simulink model "hdv_hydroelectropowertrain_model"  (R2026a)
settings: Solver=ode1be  StopTime=simulation_length  FixedStep=tsample  MaxStep=tsample
undefined symbols (not defined in the file): alpha, Apump, available_torque, Bpump, btheta_shaft, C1, consumption, Cpump, dp_lim, E0, E1, E2, E3, E_1, Elog, eta_v_m, eta_v_p, ki_dp_comp, ki_te_comp, kp_ctrl_m, kp_dp_comp, kp_te_comp, Kpump, load_blade_enable, Lpump, M, magnitude, Ncell, Npump, omega_e_rpm_ref, omega_l_max_rpm, q1Kalman, q2Kalman, q3Kalman, Qhr, R0, R1, R_tg, rKalman, rpm_base, rpm_consumption, simulation_length, tau_load, tau_load_max, Tc, torque_base, torque_consumption, torque_friction_base, tsample, v_track1_ref, v_track2_ref, valve_mmorifice_max, xv_m_max
libraries: fl_lib x383, nesl_utility x162, linear_swashplate_ctrl_lib x8, flexshaft_lib x5, bichamber_piston_lib x5, variable_displacement_motor_lib x4, variable_displacement_pump_lib x4, fixed_displacement_pump_lib x4, relief_valve_lib x4, inverse_shuttle_valve_lib x4, hydrostatic_threeway_valve_bichamber_piston_lib x4, hydrostatic_fourway_valve_bichamber_piston_lib x4
(part 7 of 8)

== system hdv_hydroelectropowertrain_model/PR776_powertrain/Hydrostatic_powertrain/driveine_RD1/vd_ctrl_pump_RD/hose3 ==
  Constant Area Hydraulic Orifice : fl_lib/Hydraulic/Hydraulic Elements/Constant Area Hydraulic Orifice  area=1e-8 m^2  C_d=0.7  lam_spec=1  B_lam=0.999  Re_cr=12  q_specify=off  q_priority=None  q=0.001 m^3/s  q_nominal_specify=off  q_nominal_value=1  q_nominal_unit=m^3/s  p_specify=off  p_priority=None  p=0 Pa  p_nominal_specify=off  p_nominal_value=1  p_nominal_unit=Pa
  Constant Area Hydraulic Orifice1 : fl_lib/Hydraulic/Hydraulic Elements/Constant Area Hydraulic Orifice  area=1e-8 m^2  C_d=0.7  lam_spec=1  B_lam=0.999  Re_cr=12  q_specify=off  q_priority=None  q=0.001 m^3/s  q_nominal_specify=off  q_nominal_value=1  q_nominal_unit=m^3/s  p_specify=off  p_priority=None  p=0 Pa  p_nominal_specify=off  p_nominal_value=1  p_nominal_unit=Pa
  Hydraulic Flow Rate Sensor3 : fl_lib/Hydraulic/Hydraulic Sensors/Hydraulic Flow Rate Sensor
  Hydraulic Flow Rate Source : fl_lib/Hydraulic/Hydraulic Sources/Hydraulic Flow Rate Source
  Hydraulic Pressure Sensor2 : fl_lib/Hydraulic/Hydraulic Sensors/Hydraulic Pressure Sensor
  Hydraulic Pressure Source : fl_lib/Hydraulic/Hydraulic Sources/Hydraulic Pressure Source
  Hydraulic Reference : fl_lib/Hydraulic/Hydraulic Elements/Hydraulic Reference
  PS Gain : fl_lib/Physical Signals/Functions/PS Gain  gain=1 Pa
  PS Gain1 : fl_lib/Physical Signals/Functions/PS Gain  gain=1 Pa^-1
  PS Gain2 : fl_lib/Physical Signals/Functions/PS Gain  gain=1 m^3/s
  PS Gain3 : fl_lib/Physical Signals/Functions/PS Gain  gain=1 m^-3*s
  PS Transfer Function : fl_lib/Physical Signals/Linear Operators/PS Transfer Function  transfer_function_type=foundation.enum.transfer_function_type.lag  T=0.01 s  T1=2 s  T2=1 s  reset_method=foundation.enum.IntegratorResetSpec.None  initial_condition_spec=foundation.enum.IntegratorICSpec.Internal  y0=0
  PS Transfer Function1 : fl_lib/Physical Signals/Linear Operators/PS Transfer Function  transfer_function_type=foundation.enum.transfer_function_type.lag  T=0.01 s  T1=2 s  T2=1 s  reset_method=foundation.enum.IntegratorResetSpec.None  initial_condition_spec=foundation.enum.IntegratorICSpec.Internal  y0=0
  A : PMIOPort  Side=Left
  AA : PMIOPort  Port=2  Side=Right
  B : PMIOPort  Port=3  Side=Left
  BB : PMIOPort  Port=4  Side=Right
  connections:
  AA/RConn1 -- Constant Area Hydraulic Orifice1/LConn1 -- Hydraulic Flow Rate Sensor3/RConn2
  PS Gain2/RConn1 -- Hydraulic Flow Rate Source/RConn1
  Hydraulic Flow Rate Sensor3/RConn1 -- PS Gain3/LConn1
  Hydraulic Flow Rate Sensor3/LConn1 -- Hydraulic Pressure Source/LConn1
  Hydraulic Pressure Source/RConn1 -- PS Gain/RConn1
  PS Gain1/LConn1 -- Hydraulic Pressure Sensor2/RConn2
  Hydraulic Pressure Source/RConn2 -- Hydraulic Pressure Sensor2/RConn1 -- Constant Area Hydraulic Orifice/RConn1 -- B/RConn1 -- Hydraulic Flow Rate Source/LConn1 -- Constant Area Hydraulic Orifice1/RConn1 -- Hydraulic Reference/LConn1 -- BB/RConn1
  PS Transfer Function1/RConn1 -- PS Gain2/LConn1
  PS Transfer Function/RConn1 -- PS Gain/LConn1
  A/RConn1 -- Constant Area Hydraulic Orifice/LConn1 -- Hydraulic Pressure Sensor2/LConn1 -- Hydraulic Flow Rate Source/RConn2
  PS Gain3/RConn1 -- PS Transfer Function1/LConn1
  PS Gain1/RConn1 -- PS Transfer Function/LConn1

== system hdv_hydroelectropowertrain_model/PR776_powertrain/Hydrostatic_powertrain/driveine_RD1/vd_ctrl_pump_RD/servo pump RD ==
  displacement reference pu : Inport
  Gain : Gain  Gain=0.03647/2
  PS Gain : fl_lib/Physical Signals/Functions/PS Gain  gain=1/(0.03647/2) m^-1
  PS-Simulink Converter7 : nesl_utility/PS-Simulink Converter  PhysicalDomain=network_engine_domain  SubClassName=ps_output  LeftPortType=input  RightPortType=output  PseudoPeriodic=off  Frequencies=[]  VectorFormat=1-D array  Unit=1  AffineConversion=off
  hydrostatic_fourway_valve_bichamber : hydrostatic_fourway_valve_bichamber_piston_lib/hydrostatic_fourway_valve_bichamber  D1=D1 m  D2=D2 m  Lp=Lp m  xv_max=xv_max mm  mp=mp kg  kp=kp N/m  bp=bp N/(m/s)  q1_specify=off  q1_priority=None  q1=0 m^3/s  q1_nominal_specify=off  q1_nominal_unit=m^3/s  q1_nominal_value=1  q2_specify=off  q2_priority=None  q2=0 m^3/s  q2_nominal_specify=off  q2_nominal_unit=m^3/s  q2_nominal_value=1  qin_specify=off  qin_priority=None  qin=0 m^3/s  qin_nominal_specify=off  qin_nominal_unit=m^3/s  qin_nominal_value=1  qout_specify=off  qout_priority=None  qout=0 m^3/s  qout_nominal_specify=off  qout_nominal_unit=m^3/s  qout_nominal_value=1  p1_specify=off  p1_priority=High  p1=125 bar  p1_nominal_specify=off  p1_nominal_unit=bar  p1_nominal_value=1  p2_specify=off  p2_priority=High  p2=125 bar  p2_nominal_specify=off  p2_nominal_unit=bar  p2_nominal_value=1  fp_specify=off  fp_priority=None  fp=0 N  fp_nominal_specify=off  fp_nominal_unit=N  fp_nominal_value=1  vp_specify=off  vp_priority=None  vp=0 m/s  vp_nominal_specify=off  vp_nominal_unit=m/s  vp_nominal_value=1  xp_specify=off  xp_priority=High  xp=500 mm  xp_nominal_specify=off  xp_nominal_unit=mm  xp_nominal_value=1
  pmlinear_actuator : pm_linear_actuator_lib/pmlinear_actuator  Bm=1 s*V/m^2  mv=mv kg  Lc=Lc H  Rc=Rc Ohm  bv=bv N/(m/s)  h=h m  xv_max=xv_max mm  n=n  ic_specify=off  ic_priority=High  ic=0 A  ic_nominal_specify=off  ic_nominal_unit=A  ic_nominal_value=1  vv_specify=off  vv_priority=None  vv=0 m/s  vv_nominal_specify=off  vv_nominal_unit=m/s  vv_nominal_value=1  xv_specify=off  xv_priority=None  xv=0 m  xv_nominal_specify=off  xv_nominal_unit=m  xv_nominal_value=1
  servo_ctrl : Subsystem
  pS : PMIOPort  Side=Left
  pT : PMIOPort  Port=2  Side=Left
  vd pu : PMIOPort  Port=3  Side=Right
  wires:
  Gain/1 -> servo_ctrl/1(ref)
  PS-Simulink Converter7/1 -> servo_ctrl/2(xp)  "xp"
  displacement reference pu/1 -> Gain/1
  connections:
  hydrostatic_fourway_valve_bichamber/LConn3 -- pT/RConn1
  hydrostatic_fourway_valve_bichamber/LConn2 -- pS/RConn1
  hydrostatic_fourway_valve_bichamber/RConn2 -- PS Gain/LConn1 -- PS-Simulink Converter7/LConn1
  servo_ctrl/RConn1 -- pmlinear_actuator/LConn1
  pmlinear_actuator/RConn1 -- hydrostatic_fourway_valve_bichamber/LConn1
  PS Gain/RConn1 -- vd pu/RConn1

== system hdv_hydroelectropowertrain_model/PR776_powertrain/Hydrostatic_powertrain/driveline_RD2/pressure_charge_system_RD/Subsystem ==
  Fixed displacement pump : fixed_displacement_pump_lib/Fixed displacement pump  max_Dv=27 cm^3/rev  inertia_pump=0.05 kg*m^2  oil_vol=2.0 l  bp=0.0025 N*m/(rad/s)  lk=1e-6 m  t_specify=off  t_priority=None  t=0 N*m  t_nominal_specify=off  t_nominal_unit=N*m  t_nominal_value=1  q_specify=off  q_priority=None  q=0 m^3/s  q_nominal_specify=off  q_nominal_unit=m^3/s  q_nominal_value=1  qt_specify=off  qt_priority=None  qt=0 m^3/s  qt_nominal_specify=off  qt_nominal_unit=m^3/s  qt_nominal_value=1  qleak_specify=off  qleak_priority=None  qleak=0 m^3/s  qleak_nominal_specify=off  qleak_nominal_unit=m^3/s  qleak_nominal_value=1  Dv_specify=off  Dv_priority=None  Dv=0 cm^3  Dv_nominal_specify=off  Dv_nominal_unit=cm^3  Dv_nominal_value=1  dp_specify=off  dp_priority=None  dp=0 Pa  dp_nominal_specify=off  dp_nominal_unit=Pa  dp_nominal_value=1  we_specify=off  we_priority=None  we=0 rad/s  we_nominal_specify=off  we_nominal_unit=rad/s  we_nominal_value=1
  Hydraulic Reference3 : fl_lib/Hydraulic/Hydraulic Elements/Hydraulic Reference
  Hydraulic Reference4 : fl_lib/Hydraulic/Hydraulic Elements/Hydraulic Reference
  relief valve : relief_valve_lib/relief valve  dp_ref=32 bar  pnom=32 bar  p_set=32 bar  p_reg=12 bar  x_rv_max=12.0 mm  qA_specify=off  qA_priority=None  qA=0 m^3/s  qA_nominal_specify=off  qA_nominal_value=1  qA_nominal_unit=m^3/s  qB_specify=off  qB_priority=None  qB=0 m^3/s  qB_nominal_specify=off  qB_nominal_value=1  qB_nominal_unit=m^3/s  dp_specify=off  dp_priority=None  dp=0 Pa  dp_nominal_specify=off  dp_nominal_value=1  dp_nominal_unit=Pa  x_rv_specify=off  x_rv_priority=None  x_rv=0 m  x_rv_nominal_specify=off  x_rv_nominal_value=1  x_rv_nominal_unit=m  x_rv_flt_specify=off  x_rv_flt_priority=None  x_rv_flt=0 m  x_rv_flt_nominal_specify=off  x_rv_flt_nominal_value=1  x_rv_flt_nominal_unit=m
      settings: LogSimulationData=on
  ps : PMIOPort  Side=Right
  D : PMIOPort  Port=2  Side=Left
  connections:
  Fixed displacement pump/LConn1 -- D/RConn1
  Fixed displacement pump/RConn2 -- Hydraulic Reference3/LConn1
  Hydraulic Reference4/LConn1 -- relief valve/RConn1
  relief valve/LConn1 -- ps/RConn1 -- Fixed displacement pump/RConn1

== system hdv_hydroelectropowertrain_model/PR776_powertrain/Hydrostatic_powertrain/driveline_RD2/pressure_charge_system_RD/hydro_check_valve1 ==
  Constant Area Hydraulic Orifice5 : fl_lib/Hydraulic/Hydraulic Elements/Constant Area Hydraulic Orifice  area=1e-4 mm^2  C_d=1  lam_spec=1  B_lam=0.999  Re_cr=12  q_specify=off  q_priority=None  q=0.001 m^3/s  q_nominal_specify=off  q_nominal_value=1  q_nominal_unit=m^3/s  p_specify=off  p_priority=None  p=0 Pa  p_nominal_specify=off  p_nominal_value=1  p_nominal_unit=Pa
  Constant Area Hydraulic Orifice6 : fl_lib/Hydraulic/Hydraulic Elements/Constant Area Hydraulic Orifice  area=4 mm^2  C_d=1  lam_spec=1  B_lam=0.999  Re_cr=12  q_specify=off  q_priority=None  q=0.001 m^3/s  q_nominal_specify=off  q_nominal_value=1  q_nominal_unit=m^3/s  p_specify=off  p_priority=None  p=0 Pa  p_nominal_specify=off  p_nominal_value=1  p_nominal_unit=Pa
  Hydraulic Flow Rate Sensor : fl_lib/Hydraulic/Hydraulic Sensors/Hydraulic Flow Rate Sensor
  Hydraulic Flow Rate Source : fl_lib/Hydraulic/Hydraulic Sources/Hydraulic Flow Rate Source
  Hydraulic Pressure Sensor : fl_lib/Hydraulic/Hydraulic Sensors/Hydraulic Pressure Sensor
  Hydraulic Pressure Source2 : fl_lib/Hydraulic/Hydraulic Sources/Hydraulic Pressure Source
  Hydraulic Reference : fl_lib/Hydraulic/Hydraulic Elements/Hydraulic Reference
  PS Saturation : fl_lib/Physical Signals/Nonlinear Operators/PS Saturation  upper_limit=inf m^3/s  lower_limit=0 m^3/s  ZeroCross=true
  PS Saturation1 : fl_lib/Physical Signals/Nonlinear Operators/PS Saturation  upper_limit=inf Pa  lower_limit=0 Pa  ZeroCross=true
  PS Transfer Function : fl_lib/Physical Signals/Linear Operators/PS Transfer Function  transfer_function_type=foundation.enum.transfer_function_type.lag  T=tsample s  T1=2 s  T2=1 s  reset_method=foundation.enum.IntegratorResetSpec.None  initial_condition_spec=foundation.enum.IntegratorICSpec.Internal  y0=0 m^3/s
  PS Transfer Function1 : fl_lib/Physical Signals/Linear Operators/PS Transfer Function  transfer_function_type=foundation.enum.transfer_function_type.lag  T=tsample s  T1=2 s  T2=1 s  reset_method=foundation.enum.IntegratorResetSpec.None  initial_condition_spec=foundation.enum.IntegratorICSpec.Internal  y0=0 Pa
  A : PMIOPort  Side=Left
  B : PMIOPort  Port=2  Side=Right
  connections:
  PS Transfer Function/LConn1 -- PS Saturation/RConn1
  PS Saturation1/RConn1 -- PS Transfer Function1/LConn1
  PS Transfer Function/RConn1 -- Hydraulic Flow Rate Source/RConn1
  Constant Area Hydraulic Orifice5/LConn1 -- A/RConn1 -- Hydraulic Pressure Sensor/LConn1 -- Hydraulic Flow Rate Source/RConn2
  Hydraulic Pressure Sensor/RConn2 -- PS Saturation1/LConn1
  PS Transfer Function1/RConn1 -- Hydraulic Pressure Source2/RConn1
  PS Saturation/LConn1 -- Hydraulic Flow Rate Sensor/RConn1
  B/RConn1 -- Constant Area Hydraulic Orifice5/RConn1 -- Hydraulic Pressure Sensor/RConn1 -- Hydraulic Flow Rate Source/LConn1
  Hydraulic Pressure Source2/LConn1 -- Hydraulic Flow Rate Sensor/LConn1
  Hydraulic Pressure Source2/RConn2 -- Hydraulic Reference/LConn1 -- Constant Area Hydraulic Orifice6/RConn1
  Hydraulic Flow Rate Sensor/RConn2 -- Constant Area Hydraulic Orifice6/LConn1

== system hdv_hydroelectropowertrain_model/PR776_powertrain/Hydrostatic_powertrain/driveline_RD2/pressure_charge_system_RD/hydro_check_valve2 ==
  Constant Area Hydraulic Orifice5 : fl_lib/Hydraulic/Hydraulic Elements/Constant Area Hydraulic Orifice  area=1e-4 mm^2  C_d=1  lam_spec=1  B_lam=0.999  Re_cr=12  q_specify=off  q_priority=None  q=0.001 m^3/s  q_nominal_specify=off  q_nominal_value=1  q_nominal_unit=m^3/s  p_specify=off  p_priority=None  p=0 Pa  p_nominal_specify=off  p_nominal_value=1  p_nominal_unit=Pa
  Constant Area Hydraulic Orifice6 : fl_lib/Hydraulic/Hydraulic Elements/Constant Area Hydraulic Orifice  area=4 mm^2  C_d=1  lam_spec=1  B_lam=0.999  Re_cr=12  q_specify=off  q_priority=None  q=0.001 m^3/s  q_nominal_specify=off  q_nominal_value=1  q_nominal_unit=m^3/s  p_specify=off  p_priority=None  p=0 Pa  p_nominal_specify=off  p_nominal_value=1  p_nominal_unit=Pa
  Hydraulic Flow Rate Sensor : fl_lib/Hydraulic/Hydraulic Sensors/Hydraulic Flow Rate Sensor
  Hydraulic Flow Rate Source : fl_lib/Hydraulic/Hydraulic Sources/Hydraulic Flow Rate Source
  Hydraulic Pressure Sensor : fl_lib/Hydraulic/Hydraulic Sensors/Hydraulic Pressure Sensor
  Hydraulic Pressure Source2 : fl_lib/Hydraulic/Hydraulic Sources/Hydraulic Pressure Source
  Hydraulic Reference : fl_lib/Hydraulic/Hydraulic Elements/Hydraulic Reference
  PS Saturation : fl_lib/Physical Signals/Nonlinear Operators/PS Saturation  upper_limit=inf m^3/s  lower_limit=0 m^3/s  ZeroCross=true
  PS Saturation1 : fl_lib/Physical Signals/Nonlinear Operators/PS Saturation  upper_limit=inf Pa  lower_limit=0 Pa  ZeroCross=true
  PS Transfer Function : fl_lib/Physical Signals/Linear Operators/PS Transfer Function  transfer_function_type=foundation.enum.transfer_function_type.lag  T=tsample s  T1=2 s  T2=1 s  reset_method=foundation.enum.IntegratorResetSpec.None  initial_condition_spec=foundation.enum.IntegratorICSpec.Internal  y0=0 m^3/s
  PS Transfer Function1 : fl_lib/Physical Signals/Linear Operators/PS Transfer Function  transfer_function_type=foundation.enum.transfer_function_type.lag  T=tsample s  T1=2 s  T2=1 s  reset_method=foundation.enum.IntegratorResetSpec.None  initial_condition_spec=foundation.enum.IntegratorICSpec.Internal  y0=0 Pa
  A : PMIOPort  Side=Left
  B : PMIOPort  Port=2  Side=Right
  connections:
  Hydraulic Flow Rate Sensor/RConn2 -- Constant Area Hydraulic Orifice6/LConn1
  Constant Area Hydraulic Orifice6/RConn1 -- Hydraulic Reference/LConn1 -- Hydraulic Pressure Source2/RConn2
  Hydraulic Pressure Source2/LConn1 -- Hydraulic Flow Rate Sensor/LConn1
  Hydraulic Flow Rate Source/LConn1 -- Hydraulic Pressure Sensor/RConn1 -- Constant Area Hydraulic Orifice5/RConn1 -- B/RConn1
  PS Saturation/LConn1 -- Hydraulic Flow Rate Sensor/RConn1
  PS Transfer Function1/RConn1 -- Hydraulic Pressure Source2/RConn1
  Hydraulic Pressure Sensor/RConn2 -- PS Saturation1/LConn1
  Hydraulic Flow Rate Source/RConn2 -- Hydraulic Pressure Sensor/LConn1 -- A/RConn1 -- Constant Area Hydraulic Orifice5/LConn1
  PS Transfer Function/RConn1 -- Hydraulic Flow Rate Source/RConn1
  PS Saturation1/RConn1 -- PS Transfer Function1/LConn1
  PS Transfer Function/LConn1 -- PS Saturation/RConn1

== system hdv_hydroelectropowertrain_model/PR776_powertrain/Hydrostatic_powertrain/driveline_RD2/vd_ctrl_motor_RD/hose3 ==
  Constant Area Hydraulic Orifice : fl_lib/Hydraulic/Hydraulic Elements/Constant Area Hydraulic Orifice  area=1e-8 m^2  C_d=0.7  lam_spec=1  B_lam=0.999  Re_cr=12  q_specify=off  q_priority=None  q=0.001 m^3/s  q_nominal_specify=off  q_nominal_value=1  q_nominal_unit=m^3/s  p_specify=off  p_priority=None  p=0 Pa  p_nominal_specify=off  p_nominal_value=1  p_nominal_unit=Pa
  Constant Area Hydraulic Orifice1 : fl_lib/Hydraulic/Hydraulic Elements/Constant Area Hydraulic Orifice  area=1e-8 m^2  C_d=0.7  lam_spec=1  B_lam=0.999  Re_cr=12  q_specify=off  q_priority=None  q=0.001 m^3/s  q_nominal_specify=off  q_nominal_value=1  q_nominal_unit=m^3/s  p_specify=off  p_priority=None  p=0 Pa  p_nominal_specify=off  p_nominal_value=1  p_nominal_unit=Pa
  Hydraulic Flow Rate Sensor3 : fl_lib/Hydraulic/Hydraulic Sensors/Hydraulic Flow Rate Sensor
  Hydraulic Flow Rate Source : fl_lib/Hydraulic/Hydraulic Sources/Hydraulic Flow Rate Source
  Hydraulic Pressure Sensor2 : fl_lib/Hydraulic/Hydraulic Sensors/Hydraulic Pressure Sensor
  Hydraulic Pressure Source : fl_lib/Hydraulic/Hydraulic Sources/Hydraulic Pressure Source
  Hydraulic Reference : fl_lib/Hydraulic/Hydraulic Elements/Hydraulic Reference
  PS Gain : fl_lib/Physical Signals/Functions/PS Gain  gain=1 Pa
  PS Gain1 : fl_lib/Physical Signals/Functions/PS Gain  gain=1 Pa^-1
  PS Gain2 : fl_lib/Physical Signals/Functions/PS Gain  gain=1 m^3/s
  PS Gain3 : fl_lib/Physical Signals/Functions/PS Gain  gain=1 m^-3*s
  PS Transfer Function : fl_lib/Physical Signals/Linear Operators/PS Transfer Function  transfer_function_type=foundation.enum.transfer_function_type.lag  T=0.01 s  T1=2 s  T2=1 s  reset_method=foundation.enum.IntegratorResetSpec.None  initial_condition_spec=foundation.enum.IntegratorICSpec.Internal  y0=0
  PS Transfer Function1 : fl_lib/Physical Signals/Linear Operators/PS Transfer Function  transfer_function_type=foundation.enum.transfer_function_type.lag  T=0.01 s  T1=2 s  T2=1 s  reset_method=foundation.enum.IntegratorResetSpec.None  initial_condition_spec=foundation.enum.IntegratorICSpec.Internal  y0=0
  A : PMIOPort  Side=Left
  AA : PMIOPort  Port=2  Side=Right
  B : PMIOPort  Port=3  Side=Left
  BB : PMIOPort  Port=4  Side=Right
  connections:
  PS Gain1/RConn1 -- PS Transfer Function/LConn1
  PS Gain3/RConn1 -- PS Transfer Function1/LConn1
  Hydraulic Flow Rate Source/RConn2 -- Hydraulic Pressure Sensor2/LConn1 -- Constant Area Hydraulic Orifice/LConn1 -- A/RConn1
  PS Transfer Function/RConn1 -- PS Gain/LConn1
  PS Transfer Function1/RConn1 -- PS Gain2/LConn1
  BB/RConn1 -- Hydraulic Reference/LConn1 -- Constant Area Hydraulic Orifice1/RConn1 -- Hydraulic Flow Rate Source/LConn1 -- B/RConn1 -- Constant Area Hydraulic Orifice/RConn1 -- Hydraulic Pressure Sensor2/RConn1 -- Hydraulic Pressure Source/RConn2
  PS Gain1/LConn1 -- Hydraulic Pressure Sensor2/RConn2
  Hydraulic Pressure Source/RConn1 -- PS Gain/RConn1
  Hydraulic Flow Rate Sensor3/LConn1 -- Hydraulic Pressure Source/LConn1
  Hydraulic Flow Rate Sensor3/RConn1 -- PS Gain3/LConn1
  PS Gain2/RConn1 -- Hydraulic Flow Rate Source/RConn1
  Hydraulic Flow Rate Sensor3/RConn2 -- Constant Area Hydraulic Orifice1/LConn1 -- AA/RConn1

== system hdv_hydroelectropowertrain_model/PR776_powertrain/Hydrostatic_powertrain/driveline_RD2/vd_ctrl_motor_RD/servo motor LD ==
  displacement reference pu : Inport
  PS Add : fl_lib/Physical Signals/Functions/PS Add
  PS Constant : fl_lib/Physical Signals/Sources/PS Constant  constant=1
  PS Gain : fl_lib/Physical Signals/Functions/PS Gain  gain=-1/0.06 m^-1
  hydrostatic_threeway_valve_bichamber_piston : hydrostatic_threeway_valve_bichamber_piston_lib/hydrostatic_threeway_valve_bichamber_piston  Dh=Dh m  Dr=Dr m  Lp=Lpm m  xv_max=xv_m_max mm  mp=mp_m kg  kp=kp_m N/m  bp=bp_m N/(m/s)  qs_specify=off  qs_priority=None  qs=0 m^3/s  qs_nominal_specify=off  qs_nominal_unit=m^3/s  qs_nominal_value=1  qv_specify=off  qv_priority=None  qv=0 m^3/s  qv_nominal_specify=off  qv_nominal_unit=m^3/s  qv_nominal_value=1  q_specify=off  q_priority=None  q=0 m^3/s  q_nominal_specify=off  q_nominal_unit=m^3/s  q_nominal_value=1  q_leak_specify=off  q_leak_priority=None  q_leak=0 m^3/s  q_leak_nominal_specify=off  q_leak_nominal_unit=m^3/s  q_leak_nominal_value=1  pc_specify=off  pc_priority=None  pc=0 bar  pc_nominal_specify=off  pc_nominal_unit=bar  pc_nominal_value=1  fp_specify=off  fp_priority=None  fp=0 N  fp_nominal_specify=off  fp_nominal_unit=N  fp_nominal_value=1  vp_specify=off  vp_priority=None  vp=0 m/s  vp_nominal_specify=off  vp_nominal_unit=m/s  vp_nominal_value=1  xp_specify=off  xp_priority=High  xp=10 mm  xp_nominal_specify=off  xp_nominal_unit=mm  xp_nominal_value=1
  servo_ctrl : Subsystem
  pS : PMIOPort  Side=Left
  pT : PMIOPort  Port=2  Side=Left
  vd : PMIOPort  Port=3  Side=Right
  wires:
  displacement reference pu/1 -> servo_ctrl/1(ref)
  connections:
  PS Constant/RConn1 -- PS Add/LConn2
  PS Gain/RConn1 -- PS Add/LConn1
  vd/RConn1 -- PS Add/RConn1
  hydrostatic_threeway_valve_bichamber_piston/LConn1 -- servo_ctrl/RConn1
  servo_ctrl/LConn1 -- PS Gain/LConn1 -- hydrostatic_threeway_valve_bichamber_piston/RConn2
  hydrostatic_threeway_valve_bichamber_piston/LConn2 -- pS/RConn1
  hydrostatic_threeway_valve_bichamber_piston/LConn3 -- pT/RConn1

== system hdv_hydroelectropowertrain_model/PR776_powertrain/Hydrostatic_powertrain/driveline_RD2/vd_ctrl_pump_RD/hose3 ==
  Constant Area Hydraulic Orifice : fl_lib/Hydraulic/Hydraulic Elements/Constant Area Hydraulic Orifice  area=1e-8 m^2  C_d=0.7  lam_spec=1  B_lam=0.999  Re_cr=12  q_specify=off  q_priority=None  q=0.001 m^3/s  q_nominal_specify=off  q_nominal_value=1  q_nominal_unit=m^3/s  p_specify=off  p_priority=None  p=0 Pa  p_nominal_specify=off  p_nominal_value=1  p_nominal_unit=Pa
  Constant Area Hydraulic Orifice1 : fl_lib/Hydraulic/Hydraulic Elements/Constant Area Hydraulic Orifice  area=1e-8 m^2  C_d=0.7  lam_spec=1  B_lam=0.999  Re_cr=12  q_specify=off  q_priority=None  q=0.001 m^3/s  q_nominal_specify=off  q_nominal_value=1  q_nominal_unit=m^3/s  p_specify=off  p_priority=None  p=0 Pa  p_nominal_specify=off  p_nominal_value=1  p_nominal_unit=Pa
  Hydraulic Flow Rate Sensor3 : fl_lib/Hydraulic/Hydraulic Sensors/Hydraulic Flow Rate Sensor
  Hydraulic Flow Rate Source : fl_lib/Hydraulic/Hydraulic Sources/Hydraulic Flow Rate Source
  Hydraulic Pressure Sensor2 : fl_lib/Hydraulic/Hydraulic Sensors/Hydraulic Pressure Sensor
  Hydraulic Pressure Source : fl_lib/Hydraulic/Hydraulic Sources/Hydraulic Pressure Source
  Hydraulic Reference : fl_lib/Hydraulic/Hydraulic Elements/Hydraulic Reference
  PS Gain : fl_lib/Physical Signals/Functions/PS Gain  gain=1 Pa
  PS Gain1 : fl_lib/Physical Signals/Functions/PS Gain  gain=1 Pa^-1
  PS Gain2 : fl_lib/Physical Signals/Functions/PS Gain  gain=1 m^3/s
  PS Gain3 : fl_lib/Physical Signals/Functions/PS Gain  gain=1 m^-3*s
  PS Transfer Function : fl_lib/Physical Signals/Linear Operators/PS Transfer Function  transfer_function_type=foundation.enum.transfer_function_type.lag  T=0.01 s  T1=2 s  T2=1 s  reset_method=foundation.enum.IntegratorResetSpec.None  initial_condition_spec=foundation.enum.IntegratorICSpec.Internal  y0=0
  PS Transfer Function1 : fl_lib/Physical Signals/Linear Operators/PS Transfer Function  transfer_function_type=foundation.enum.transfer_function_type.lag  T=0.01 s  T1=2 s  T2=1 s  reset_method=foundation.enum.IntegratorResetSpec.None  initial_condition_spec=foundation.enum.IntegratorICSpec.Internal  y0=0
  A : PMIOPort  Side=Left
  AA : PMIOPort  Port=2  Side=Right
  B : PMIOPort  Port=3  Side=Left
  BB : PMIOPort  Port=4  Side=Right
  connections:
  PS Gain1/RConn1 -- PS Transfer Function/LConn1
  PS Gain3/RConn1 -- PS Transfer Function1/LConn1
  Hydraulic Flow Rate Source/RConn2 -- Hydraulic Pressure Sensor2/LConn1 -- Constant Area Hydraulic Orifice/LConn1 -- A/RConn1
  PS Transfer Function/RConn1 -- PS Gain/LConn1
  PS Transfer Function1/RConn1 -- PS Gain2/LConn1
  BB/RConn1 -- Hydraulic Reference/LConn1 -- Constant Area Hydraulic Orifice1/RConn1 -- Hydraulic Flow Rate Source/LConn1 -- B/RConn1 -- Constant Area Hydraulic Orifice/RConn1 -- Hydraulic Pressure Sensor2/RConn1 -- Hydraulic Pressure Source/RConn2
  PS Gain1/LConn1 -- Hydraulic Pressure Sensor2/RConn2
  Hydraulic Pressure Source/RConn1 -- PS Gain/RConn1
  Hydraulic Flow Rate Sensor3/LConn1 -- Hydraulic Pressure Source/LConn1
  Hydraulic Flow Rate Sensor3/RConn1 -- PS Gain3/LConn1
  PS Gain2/RConn1 -- Hydraulic Flow Rate Source/RConn1
  Hydraulic Flow Rate Sensor3/RConn2 -- Constant Area Hydraulic Orifice1/LConn1 -- AA/RConn1

== system hdv_hydroelectropowertrain_model/PR776_powertrain/Hydrostatic_powertrain/driveline_RD2/vd_ctrl_pump_RD/servo pump RD ==
  displacement reference pu : Inport
  Gain : Gain  Gain=0.03647/2
  PS Gain : fl_lib/Physical Signals/Functions/PS Gain  gain=1/(0.03647/2) m^-1
  PS-Simulink Converter7 : nesl_utility/PS-Simulink Converter  PhysicalDomain=network_engine_domain  SubClassName=ps_output  LeftPortType=input  RightPortType=output  PseudoPeriodic=off  Frequencies=[]  VectorFormat=1-D array  Unit=1  AffineConversion=off
  hydrostatic_fourway_valve_bichamber : hydrostatic_fourway_valve_bichamber_piston_lib/hydrostatic_fourway_valve_bichamber  D1=D1 m  D2=D2 m  Lp=Lp m  xv_max=xv_max mm  mp=mp kg  kp=kp N/m  bp=bp N/(m/s)  q1_specify=off  q1_priority=None  q1=0 m^3/s  q1_nominal_specify=off  q1_nominal_unit=m^3/s  q1_nominal_value=1  q2_specify=off  q2_priority=None  q2=0 m^3/s  q2_nominal_specify=off  q2_nominal_unit=m^3/s  q2_nominal_value=1  qin_specify=off  qin_priority=None  qin=0 m^3/s  qin_nominal_specify=off  qin_nominal_unit=m^3/s  qin_nominal_value=1  qout_specify=off  qout_priority=None  qout=0 m^3/s  qout_nominal_specify=off  qout_nominal_unit=m^3/s  qout_nominal_value=1  p1_specify=off  p1_priority=High  p1=125 bar  p1_nominal_specify=off  p1_nominal_unit=bar  p1_nominal_value=1  p2_specify=off  p2_priority=High  p2=125 bar  p2_nominal_specify=off  p2_nominal_unit=bar  p2_nominal_value=1  fp_specify=off  fp_priority=None  fp=0 N  fp_nominal_specify=off  fp_nominal_unit=N  fp_nominal_value=1  vp_specify=off  vp_priority=None  vp=0 m/s  vp_nominal_specify=off  vp_nominal_unit=m/s  vp_nominal_value=1  xp_specify=off  xp_priority=High  xp=500 mm  xp_nominal_specify=off  xp_nominal_unit=mm  xp_nominal_value=1
  pmlinear_actuator : pm_linear_actuator_lib/pmlinear_actuator  Bm=1 s*V/m^2  mv=mv kg  Lc=Lc H  Rc=Rc Ohm  bv=bv N/(m/s)  h=h m  xv_max=xv_max mm  n=n  ic_specify=off  ic_priority=High  ic=0 A  ic_nominal_specify=off  ic_nominal_unit=A  ic_nominal_value=1  vv_specify=off  vv_priority=None  vv=0 m/s  vv_nominal_specify=off  vv_nominal_unit=m/s  vv_nominal_value=1  xv_specify=off  xv_priority=None  xv=0 m  xv_nominal_specify=off  xv_nominal_unit=m  xv_nominal_value=1
  servo_ctrl : Subsystem
  pS : PMIOPort  Side=Left
  pT : PMIOPort  Port=2  Side=Left
  vd pu : PMIOPort  Port=3  Side=Right
  wires:
  displacement reference pu/1 -> Gain/1
  PS-Simulink Converter7/1 -> servo_ctrl/2(xp)  "xp"
  Gain/1 -> servo_ctrl/1(ref)
  connections:
  PS Gain/RConn1 -- vd pu/RConn1
  pmlinear_actuator/RConn1 -- hydrostatic_fourway_valve_bichamber/LConn1
  servo_ctrl/RConn1 -- pmlinear_actuator/LConn1
  PS-Simulink Converter7/LConn1 -- PS Gain/LConn1 -- hydrostatic_fourway_valve_bichamber/RConn2
  hydrostatic_fourway_valve_bichamber/LConn2 -- pS/RConn1
  hydrostatic_fourway_valve_bichamber/LConn3 -- pT/RConn1

== system hdv_hydroelectropowertrain_model/PR776_powertrain/electrical_main_drive_train/dc//dc/iin_ref/current_reference ==
  Constant1 : Constant  Value=250
  iin_ref : Outport
  wires:
  Constant1/1 -> iin_ref/1

== system hdv_hydroelectropowertrain_model/PR776_powertrain/electrical_main_drive_train/dc//dc/iout_ref/current_reference ==
  Constant1 : Constant  Value=350
  Manual Switch : ManualSwitch
  Rate Limiter2 : RateLimiter  RisingSlewLimit=500  FallingSlewLimit=-500  SampleTimeMode=inherited
  Step2 : Step  Time=simulation_length*3/5  InitialValue=55e3/760  FinalValue=8e3/760  SampleTime=0
  Transfer Fcn1 : TransferFcn  Denominator=[1e-1 1]
  iout_ref : Outport
  wires:
  Step2/1 -> Rate Limiter2/1
  Rate Limiter2/1 -> Transfer Fcn1/1
  Constant1/1 -> Manual Switch/1
  Manual Switch/1 -> iout_ref/1
  Transfer Fcn1/1 -> Manual Switch/2

== system hdv_hydroelectropowertrain_model/PR776_powertrain/electrical_main_drive_train/dc//dc/vi ctrl/Iin Ctrl ==
  iin_ref : Inport
  iin : Inport  Port=2
  Sum2 : Sum  Inputs=+-  OutDataTypeStr=double  AccumDataTypeStr=double  SaturateOnIntegerOverflow=on
  iin_ctrl : Subsystem
  ctrli_out : Outport
  wires:
  Sum2/1 -> iin_ctrl/1(i_tilde)
  iin_ref/1 -> Sum2/1
  iin/1 -> Sum2/2
  iin_ctrl/1(ctrli_out) -> ctrli_out/1

== system hdv_hydroelectropowertrain_model/PR776_powertrain/electrical_main_drive_train/dc//dc/vi ctrl/Iout Ctrl ==
  iout_ref : Inport
  iout : Inport  Port=2
  Sum2 : Sum  Inputs=+-  OutDataTypeStr=double  AccumDataTypeStr=double  SaturateOnIntegerOverflow=on
  iout_ctrl : Subsystem
  ctrli_out : Outport
  wires:
  iout_ctrl/1(ctrli_out) -> ctrli_out/1
  iout/1 -> Sum2/2
  iout_ref/1 -> Sum2/1
  Sum2/1 -> iout_ctrl/1(i_tilde)

== system hdv_hydroelectropowertrain_model/PR776_powertrain/electrical_main_drive_train/dc//dc/vi ctrl/Vout Ctrl ==
  vout_ref : Inport
  vout : Inport  Port=2
  Sum2 : Sum  Inputs=+-  OutDataTypeStr=double  AccumDataTypeStr=double  SaturateOnIntegerOverflow=on
  vout_ctrl : Subsystem
  ctrlv_out : Outport
  wires:
  vout_ref/1 -> Sum2/1
  vout/1 -> Sum2/2
  vout_ctrl/1(ctrlv_out) -> ctrlv_out/1
  Sum2/1 -> vout_ctrl/1(ixi_tilde)

== system hdv_hydroelectropowertrain_model/PR776_powertrain/electrical_main_drive_train/dc//dc/vout_ref/voltage_reference ==
  Constant1 : Constant  Value=760
  vout_ref : Outport
  wires:
  Constant1/1 -> vout_ref/1

== system hdv_hydroelectropowertrain_model/PR776_powertrain/electrical_main_drive_train/pmsm_ctrl/pmsm_dq_ctrl/phaseU ==
  Controlled Current Source : fl_lib/Electrical/Electrical Sources/Controlled Current Source
  PS Divide : fl_lib/Physical Signals/Functions/PS Divide
  PS Saturation : fl_lib/Physical Signals/Nonlinear Operators/PS Saturation  upper_limit=inf V  lower_limit=1 V  ZeroCross=true
  Resistor : fl_lib/Electrical/Electrical Elements/Resistor  R=1e4 Ohm  i_specify=off  i_priority=None  i=0 A  i_nominal_specify=off  i_nominal_value=1  i_nominal_unit=A  v_specify=off  v_priority=None  v=0 V  v_nominal_specify=off  v_nominal_value=1  v_nominal_unit=V
  Voltage Sensor : fl_lib/Electrical/Electrical Sensors/Voltage Sensor
  pin : PMIOPort  Side=Left
  u1+ : PMIOPort  Port=2  Side=Left
  u1- : PMIOPort  Port=3  Side=Left
  connections:
  pin/RConn1 -- PS Divide/LConn1
  Voltage Sensor/LConn1 -- Resistor/LConn1 -- u1+/RConn1 -- Controlled Current Source/RConn2
  PS Saturation/RConn1 -- PS Divide/LConn2
  Voltage Sensor/RConn2 -- Resistor/RConn1 -- u1-/RConn1 -- Controlled Current Source/LConn1
  Controlled Current Source/RConn1 -- PS Divide/RConn1
  Voltage Sensor/RConn1 -- PS Saturation/LConn1

== system hdv_hydroelectropowertrain_model/PR776_powertrain/front_blade_model/piston_tilt/controller/controller ==
  ref : Inport
  xp : Inport  Port=2
  Gain : Gain  Gain=200
  Saturation : Saturate  UpperLimit=valve_mmorifice_max  LowerLimit=-valve_mmorifice_max
  Simulink-PS Converter : nesl_utility/Simulink-PS Converter  PhysicalDomain=network_engine_domain  SubClassName=ps_input  LeftPortType=input  RightPortType=output  PseudoPeriodic=off  Frequencies=[]  NoiseDistribution=none  NoiseParameters=[]  Unit=mm  AffineConversion=on  FilteringAndDerivatives=provide  SimscapeFilterOrder=2  InputFilterTimeConstant=0.025  UdotUserProvided=0
  Sum3 : Sum  Inputs=-+|
  Unit Delay : UnitDelay  SampleTime=tsample
  Unit Delay1 : UnitDelay  SampleTime=tsample
  xv : PMIOPort  Side=Right
  wires:
  Unit Delay/1 -> Sum3/2
  xp/1 -> Unit Delay1/1
  Sum3/1 -> Gain/1
  Unit Delay1/1 -> Sum3/1
  Gain/1 -> Saturation/1
  ref/1 -> Unit Delay/1
  Saturation/1 -> Simulink-PS Converter/1
  connections:
  Simulink-PS Converter/RConn1 -- xv/RConn1

== system hdv_hydroelectropowertrain_model/PR776_powertrain/front_blade_model/pistons_height/controller/controller ==
  ref : Inport
  xp : Inport  Port=2
  Gain : Gain  Gain=200
  Saturation : Saturate  UpperLimit=valve_mmorifice_max  LowerLimit=-valve_mmorifice_max
  Simulink-PS Converter : nesl_utility/Simulink-PS Converter  PhysicalDomain=network_engine_domain  SubClassName=ps_input  LeftPortType=input  RightPortType=output  PseudoPeriodic=off  Frequencies=[]  NoiseDistribution=none  NoiseParameters=[]  Unit=mm  AffineConversion=on  FilteringAndDerivatives=provide  SimscapeFilterOrder=2  InputFilterTimeConstant=0.025  UdotUserProvided=0
  Sum3 : Sum  Inputs=-+|
  Unit Delay : UnitDelay  SampleTime=tsample
  Unit Delay1 : UnitDelay  SampleTime=tsample
  xv scope : Scope
      settings: ActiveDisplayYMinimum=-0.11706  ActiveDisplayYMaximum=1.05351
  xv : PMIOPort  Side=Right
  wires:
  Sum3/1 -> Gain/1
  xp/1 -> Unit Delay1/1
  Unit Delay/1 -> Sum3/2
  Unit Delay1/1 -> Sum3/1
  ref/1 -> Unit Delay/1
  Gain/1 -> Saturation/1
  Saturation/1 -> xv scope/1, Simulink-PS Converter/1
  connections:
  Simulink-PS Converter/RConn1 -- xv/RConn1

== system hdv_hydroelectropowertrain_model/PR776_powertrain/front_blade_model/pistons_pitch/controller/controller ==
  ref : Inport
  xp : Inport  Port=2
  Gain : Gain  Gain=200
  Saturation : Saturate  UpperLimit=valve_mmorifice_max  LowerLimit=-valve_mmorifice_max
  Simulink-PS Converter : nesl_utility/Simulink-PS Converter  PhysicalDomain=network_engine_domain  SubClassName=ps_input  LeftPortType=input  RightPortType=output  PseudoPeriodic=off  Frequencies=[]  NoiseDistribution=none  NoiseParameters=[]  Unit=mm  AffineConversion=on  FilteringAndDerivatives=provide  SimscapeFilterOrder=2  InputFilterTimeConstant=0.025  UdotUserProvided=0
  Sum3 : Sum  Inputs=-+|
  Unit Delay : UnitDelay  SampleTime=tsample
  Unit Delay1 : UnitDelay  SampleTime=tsample
  xv : PMIOPort  Side=Right
  wires:
  Gain/1 -> Saturation/1
  Unit Delay1/1 -> Sum3/1
  Sum3/1 -> Gain/1
  xp/1 -> Unit Delay1/1
  Unit Delay/1 -> Sum3/2
  ref/1 -> Unit Delay/1
  Saturation/1 -> Simulink-PS Converter/1
  connections:
  Simulink-PS Converter/RConn1 -- xv/RConn1

== system hdv_hydroelectropowertrain_model/PR776_powertrain/Hydrostatic_powertrain/driveine_LD1/vd_ctrl_motor_LD/servo motor LD/servo_ctrl ==
  ref : Inport
  Constant : Constant
  Gain : Gain  Gain=0.06
  PS Gain : fl_lib/Physical Signals/Functions/PS Gain  gain=kp_ctrl_m
  PS Saturation : fl_lib/Physical Signals/Nonlinear Operators/PS Saturation  upper_limit=xv_m_max m  lower_limit=-xv_m_max m  ZeroCross=true
  PS Subtract : fl_lib/Physical Signals/Functions/PS Subtract
  Simulink-PS Converter1 : nesl_utility/Simulink-PS Converter  PhysicalDomain=network_engine_domain  SubClassName=ps_input  LeftPortType=input  RightPortType=output  PseudoPeriodic=off  Frequencies=[]  NoiseDistribution=none  NoiseParameters=[]  Unit=m  AffineConversion=on  FilteringAndDerivatives=provide  SimscapeFilterOrder=2  InputFilterTimeConstant=0.025  UdotUserProvided=0
  Sum : Sum  Inputs=|-+
  xv : PMIOPort  Side=Right
  xp : PMIOPort  Port=2  Side=Left
  wires:
  Gain/1 -> Simulink-PS Converter1/1
  Sum/1 -> Gain/1
  Constant/1 -> Sum/2
  ref/1 -> Sum/1
  connections:
  PS Saturation/RConn1 -- xv/RConn1
  PS Saturation/LConn1 -- PS Gain/RConn1
  PS Gain/LConn1 -- PS Subtract/RConn1
  xp/RConn1 -- PS Subtract/LConn2
  PS Subtract/LConn1 -- Simulink-PS Converter1/RConn1

== system hdv_hydroelectropowertrain_model/PR776_powertrain/Hydrostatic_powertrain/driveine_LD1/vd_ctrl_pump_LD/servo pump RD/servo_ctrl ==
  ref : Inport
  xp : Inport  Port=2
  Gain : Gain  Gain=Bpump  Multiplication=Matrix(K*u)
  Gain1 : Gain  Gain=Apump  Multiplication=Matrix(K*u)
  Gain2 : Gain  Gain=Cpump  Multiplication=Matrix(K*u)
  Gain3 : Gain  Gain=Lpump  Multiplication=Matrix(K*u)
  Gain4 : Gain  Gain=Kpump  Multiplication=Matrix(K*u)
  Gain6 : Gain  Gain=Npump
  Integrator : Integrator
  Simulink-PS Converter1 : nesl_utility/Simulink-PS Converter  PhysicalDomain=network_engine_domain  SubClassName=ps_input  LeftPortType=input  RightPortType=output  PseudoPeriodic=off  Frequencies=[]  NoiseDistribution=none  NoiseParameters=[]  Unit=V  AffineConversion=off  FilteringAndDerivatives=provide  SimscapeFilterOrder=2  InputFilterTimeConstant=0.025  UdotUserProvided=0
  Sum : Sum  Inputs=|++
  Sum1 : Sum  Inputs=|++
  Sum2 : Sum  Inputs=+-|
  Sum3 : Sum  Inputs=-+|
  Transfer Fcn1 : TransferFcn  Denominator=[1e-6 1]
  uc : PMIOPort  Side=Right
  wires:
  Transfer Fcn1/1 -> Sum2/1
  Gain4/1 -> Sum3/1
  Gain6/1 -> Sum3/2
  ref/1 -> Gain6/1
  Integrator/1 -> Gain1/1, Gain2/1, Gain4/1
  Sum/1 -> Sum1/1
  Gain/1 -> Sum/1
  Gain1/1 -> Sum1/2
  Gain2/1 -> Sum2/2
  Sum2/1 -> Gain3/1
  xp/1 -> Transfer Fcn1/1
  Sum1/1 -> Integrator/1
  Gain3/1 -> Sum/2
  Sum3/1 -> Simulink-PS Converter1/1, Gain/1
  connections:
  uc/RConn1 -- Simulink-PS Converter1/RConn1

== system hdv_hydroelectropowertrain_model/PR776_powertrain/Hydrostatic_powertrain/driveine_LD2/vd_ctrl_motor_LD/servo motor LD/servo_ctrl ==
  ref : Inport
  Constant : Constant
  Gain : Gain  Gain=0.06
  PS Gain : fl_lib/Physical Signals/Functions/PS Gain  gain=kp_ctrl_m
  PS Saturation : fl_lib/Physical Signals/Nonlinear Operators/PS Saturation  upper_limit=xv_m_max m  lower_limit=-xv_m_max m  ZeroCross=true
  PS Subtract : fl_lib/Physical Signals/Functions/PS Subtract
  Simulink-PS Converter1 : nesl_utility/Simulink-PS Converter  PhysicalDomain=network_engine_domain  SubClassName=ps_input  LeftPortType=input  RightPortType=output  PseudoPeriodic=off  Frequencies=[]  NoiseDistribution=none  NoiseParameters=[]  Unit=m  AffineConversion=on  FilteringAndDerivatives=provide  SimscapeFilterOrder=2  InputFilterTimeConstant=0.025  UdotUserProvided=0
  Sum : Sum  Inputs=|-+
  xv : PMIOPort  Side=Right
  xp : PMIOPort  Port=2  Side=Left
  wires:
  ref/1 -> Sum/1
  Constant/1 -> Sum/2
  Sum/1 -> Gain/1
  Gain/1 -> Simulink-PS Converter1/1
  connections:
  PS Subtract/LConn1 -- Simulink-PS Converter1/RConn1
  xp/RConn1 -- PS Subtract/LConn2
  PS Gain/LConn1 -- PS Subtract/RConn1
  PS Saturation/LConn1 -- PS Gain/RConn1
  PS Saturation/RConn1 -- xv/RConn1

== system hdv_hydroelectropowertrain_model/PR776_powertrain/Hydrostatic_powertrain/driveine_LD2/vd_ctrl_pump_LD/servo pump RD/servo_ctrl ==
  ref : Inport
  xp : Inport  Port=2
  Gain : Gain  Gain=Bpump  Multiplication=Matrix(K*u)
  Gain1 : Gain  Gain=Apump  Multiplication=Matrix(K*u)
  Gain2 : Gain  Gain=Cpump  Multiplication=Matrix(K*u)
  Gain3 : Gain  Gain=Lpump  Multiplication=Matrix(K*u)
  Gain4 : Gain  Gain=Kpump  Multiplication=Matrix(K*u)
  Gain6 : Gain  Gain=Npump
  Integrator : Integrator
  Simulink-PS Converter1 : nesl_utility/Simulink-PS Converter  PhysicalDomain=network_engine_domain  SubClassName=ps_input  LeftPortType=input  RightPortType=output  PseudoPeriodic=off  Frequencies=[]  NoiseDistribution=none  NoiseParameters=[]  Unit=V  AffineConversion=off  FilteringAndDerivatives=provide  SimscapeFilterOrder=2  InputFilterTimeConstant=0.025  UdotUserProvided=0
  Sum : Sum  Inputs=|++
  Sum1 : Sum  Inputs=|++
  Sum2 : Sum  Inputs=+-|
  Sum3 : Sum  Inputs=-+|
  Transfer Fcn1 : TransferFcn  Denominator=[1e-6 1]
  uc : PMIOPort  Side=Right
  wires:
  Sum3/1 -> Gain/1, Simulink-PS Converter1/1
  Gain3/1 -> Sum/2
  Sum1/1 -> Integrator/1
  xp/1 -> Transfer Fcn1/1
  Sum2/1 -> Gain3/1
  Gain2/1 -> Sum2/2
  Gain1/1 -> Sum1/2
  Gain/1 -> Sum/1
  Sum/1 -> Sum1/1
  Integrator/1 -> Gain4/1, Gain2/1, Gain1/1
  ref/1 -> Gain6/1
  Gain6/1 -> Sum3/2
  Gain4/1 -> Sum3/1
  Transfer Fcn1/1 -> Sum2/1
  connections:
  uc/RConn1 -- Simulink-PS Converter1/RConn1

== system hdv_hydroelectropowertrain_model/PR776_powertrain/Hydrostatic_powertrain/driveine_RD1/vd_ctrl_motor_RD/servo motor LD/servo_ctrl ==
  ref : Inport
  Constant : Constant
  Gain : Gain  Gain=0.06
  PS Gain : fl_lib/Physical Signals/Functions/PS Gain  gain=kp_ctrl_m
  PS Saturation : fl_lib/Physical Signals/Nonlinear Operators/PS Saturation  upper_limit=xv_m_max m  lower_limit=-xv_m_max m  ZeroCross=true
  PS Subtract : fl_lib/Physical Signals/Functions/PS Subtract
  Simulink-PS Converter1 : nesl_utility/Simulink-PS Converter  PhysicalDomain=network_engine_domain  SubClassName=ps_input  LeftPortType=input  RightPortType=output  PseudoPeriodic=off  Frequencies=[]  NoiseDistribution=none  NoiseParameters=[]  Unit=m  AffineConversion=on  FilteringAndDerivatives=provide  SimscapeFilterOrder=2  InputFilterTimeConstant=0.025  UdotUserProvided=0
  Sum : Sum  Inputs=|-+
  xv : PMIOPort  Side=Right
  xp : PMIOPort  Port=2  Side=Left
  wires:
  ref/1 -> Sum/1
  Constant/1 -> Sum/2
  Sum/1 -> Gain/1
  Gain/1 -> Simulink-PS Converter1/1
  connections:
  PS Subtract/LConn1 -- Simulink-PS Converter1/RConn1
  xp/RConn1 -- PS Subtract/LConn2
  PS Gain/LConn1 -- PS Subtract/RConn1
  PS Saturation/LConn1 -- PS Gain/RConn1
  xv/RConn1 -- PS Saturation/RConn1

== system hdv_hydroelectropowertrain_model/PR776_powertrain/Hydrostatic_powertrain/driveine_RD1/vd_ctrl_pump_RD/servo pump RD/servo_ctrl ==
  ref : Inport
  xp : Inport  Port=2
  Gain : Gain  Gain=Bpump  Multiplication=Matrix(K*u)
  Gain1 : Gain  Gain=Apump  Multiplication=Matrix(K*u)
  Gain2 : Gain  Gain=Cpump  Multiplication=Matrix(K*u)
  Gain3 : Gain  Gain=Lpump  Multiplication=Matrix(K*u)
  Gain4 : Gain  Gain=Kpump  Multiplication=Matrix(K*u)
  Gain6 : Gain  Gain=Npump
  Integrator : Integrator
  Simulink-PS Converter1 : nesl_utility/Simulink-PS Converter  PhysicalDomain=network_engine_domain  SubClassName=ps_input  LeftPortType=input  RightPortType=output  PseudoPeriodic=off  Frequencies=[]  NoiseDistribution=none  NoiseParameters=[]  Unit=V  AffineConversion=off  FilteringAndDerivatives=provide  SimscapeFilterOrder=2  InputFilterTimeConstant=0.025  UdotUserProvided=0
  Sum : Sum  Inputs=|++
  Sum1 : Sum  Inputs=|++
  Sum2 : Sum  Inputs=+-|
  Sum3 : Sum  Inputs=-+|
  Transfer Fcn1 : TransferFcn  Denominator=[1e-6 1]
  uc : PMIOPort  Side=Right
  wires:
  Transfer Fcn1/1 -> Sum2/1
  Gain4/1 -> Sum3/1
  Gain6/1 -> Sum3/2
  ref/1 -> Gain6/1
  Integrator/1 -> Gain1/1, Gain2/1, Gain4/1
  Sum/1 -> Sum1/1
  Gain/1 -> Sum/1
  Gain1/1 -> Sum1/2
  Gain2/1 -> Sum2/2
  Sum2/1 -> Gain3/1
  xp/1 -> Transfer Fcn1/1
  Sum1/1 -> Integrator/1
  Gain3/1 -> Sum/2
  Sum3/1 -> Simulink-PS Converter1/1, Gain/1
  connections:
  uc/RConn1 -- Simulink-PS Converter1/RConn1

== system hdv_hydroelectropowertrain_model/PR776_powertrain/Hydrostatic_powertrain/driveline_RD2/vd_ctrl_motor_RD/servo motor LD/servo_ctrl ==
  ref : Inport
  Constant : Constant
  Gain : Gain  Gain=0.06
  PS Gain : fl_lib/Physical Signals/Functions/PS Gain  gain=kp_ctrl_m
  PS Saturation : fl_lib/Physical Signals/Nonlinear Operators/PS Saturation  upper_limit=xv_m_max m  lower_limit=-xv_m_max m  ZeroCross=true
  PS Subtract : fl_lib/Physical Signals/Functions/PS Subtract
  Simulink-PS Converter1 : nesl_utility/Simulink-PS Converter  PhysicalDomain=network_engine_domain  SubClassName=ps_input  LeftPortType=input  RightPortType=output  PseudoPeriodic=off  Frequencies=[]  NoiseDistribution=none  NoiseParameters=[]  Unit=m  AffineConversion=on  FilteringAndDerivatives=provide  SimscapeFilterOrder=2  InputFilterTimeConstant=0.025  UdotUserProvided=0
  Sum : Sum  Inputs=|-+
  xv : PMIOPort  Side=Right
  xp : PMIOPort  Port=2  Side=Left
  wires:
  Gain/1 -> Simulink-PS Converter1/1
  Sum/1 -> Gain/1
  Constant/1 -> Sum/2
  ref/1 -> Sum/1
  connections:
  xv/RConn1 -- PS Saturation/RConn1
  PS Saturation/LConn1 -- PS Gain/RConn1
  PS Gain/LConn1 -- PS Subtract/RConn1
  xp/RConn1 -- PS Subtract/LConn2
  PS Subtract/LConn1 -- Simulink-PS Converter1/RConn1

== system hdv_hydroelectropowertrain_model/PR776_powertrain/Hydrostatic_powertrain/driveline_RD2/vd_ctrl_pump_RD/servo pump RD/servo_ctrl ==
  ref : Inport
  xp : Inport  Port=2
  Gain : Gain  Gain=Bpump  Multiplication=Matrix(K*u)
  Gain1 : Gain  Gain=Apump  Multiplication=Matrix(K*u)
  Gain2 : Gain  Gain=Cpump  Multiplication=Matrix(K*u)
  Gain3 : Gain  Gain=Lpump  Multiplication=Matrix(K*u)
  Gain4 : Gain  Gain=Kpump  Multiplication=Matrix(K*u)
  Gain6 : Gain  Gain=Npump
  Integrator : Integrator
  Simulink-PS Converter1 : nesl_utility/Simulink-PS Converter  PhysicalDomain=network_engine_domain  SubClassName=ps_input  LeftPortType=input  RightPortType=output  PseudoPeriodic=off  Frequencies=[]  NoiseDistribution=none  NoiseParameters=[]  Unit=V  AffineConversion=off  FilteringAndDerivatives=provide  SimscapeFilterOrder=2  InputFilterTimeConstant=0.025  UdotUserProvided=0
  Sum : Sum  Inputs=|++
  Sum1 : Sum  Inputs=|++
  Sum2 : Sum  Inputs=+-|
  Sum3 : Sum  Inputs=-+|
  Transfer Fcn1 : TransferFcn  Denominator=[1e-6 1]
  uc : PMIOPort  Side=Right
  wires:
  Sum3/1 -> Gain/1, Simulink-PS Converter1/1
  Gain3/1 -> Sum/2
  Sum1/1 -> Integrator/1
  xp/1 -> Transfer Fcn1/1
  Sum2/1 -> Gain3/1
  Gain2/1 -> Sum2/2
  Gain1/1 -> Sum1/2
  Gain/1 -> Sum/1
  Sum/1 -> Sum1/1
  Integrator/1 -> Gain4/1, Gain2/1, Gain1/1
  ref/1 -> Gain6/1
  Gain6/1 -> Sum3/2
  Gain4/1 -> Sum3/1
  Transfer Fcn1/1 -> Sum2/1
  connections:
  uc/RConn1 -- Simulink-PS Converter1/RConn1

== system hdv_hydroelectropowertrain_model/PR776_powertrain/electrical_main_drive_train/dc//dc/vi ctrl/Iin Ctrl/iin_ctrl ==
  i_tilde : Inport
  1/Ti : Gain  Gain=0.25  ParamDataTypeStr=double  OutDataTypeStr=double  SaturateOnIntegerOverflow=on
  1/Ti1 : Gain  ParamDataTypeStr=double  OutDataTypeStr=double  SaturateOnIntegerOverflow=on
  Saturation2 : Saturate  UpperLimit=12  LowerLimit=0  OutDataTypeStr=double
  Sum1 : Sum  Inputs=+++  SaturateOnIntegerOverflow=on
  Sum4 : Sum  Inputs=-+  SaturateOnIntegerOverflow=on
  Unit Delay4 : UnitDelay  SampleTime=tsample
  kp2 : Gain  Gain=18*tsample  ParamDataTypeStr=double  OutDataTypeStr=double  SaturateOnIntegerOverflow=on
  ctrli_out : Outport
  wires:
  1/Ti1/1 -> 1/Ti/1, kp2/1
  Saturation2/1 -> ctrli_out/1, Sum4/2
  Unit Delay4/1 -> Sum1/3
  Sum4/1 -> Unit Delay4/1
  1/Ti/1 -> Sum4/1, Sum1/1
  kp2/1 -> Sum1/2
  Sum1/1 -> Saturation2/1
  i_tilde/1 -> 1/Ti1/1

== system hdv_hydroelectropowertrain_model/PR776_powertrain/electrical_main_drive_train/dc//dc/vi ctrl/Iout Ctrl/iout_ctrl ==
  i_tilde : Inport
  1/Ti : Gain  Gain=0.25  ParamDataTypeStr=double  OutDataTypeStr=double  SaturateOnIntegerOverflow=on
  1/Ti1 : Gain  ParamDataTypeStr=double  OutDataTypeStr=double  SaturateOnIntegerOverflow=on
  Saturation2 : Saturate  UpperLimit=12  LowerLimit=0  OutDataTypeStr=double
  Sum1 : Sum  Inputs=+++  SaturateOnIntegerOverflow=on
  Sum4 : Sum  Inputs=-+  SaturateOnIntegerOverflow=on
  Unit Delay4 : UnitDelay  SampleTime=tsample
  kp2 : Gain  Gain=18*tsample  ParamDataTypeStr=double  OutDataTypeStr=double  SaturateOnIntegerOverflow=on
  ctrli_out : Outport
  wires:
  i_tilde/1 -> 1/Ti1/1
  Sum1/1 -> Saturation2/1
  kp2/1 -> Sum1/2
  1/Ti/1 -> Sum1/1, Sum4/1
  Sum4/1 -> Unit Delay4/1
  Unit Delay4/1 -> Sum1/3
  Saturation2/1 -> Sum4/2, ctrli_out/1
  1/Ti1/1 -> kp2/1, 1/Ti/1

== system hdv_hydroelectropowertrain_model/PR776_powertrain/electrical_main_drive_train/dc//dc/vi ctrl/Vout Ctrl/vout_ctrl ==
  ixi_tilde : Inport
  1/Ti : Gain  Gain=0.25  ParamDataTypeStr=double  OutDataTypeStr=double  SaturateOnIntegerOverflow=on
  1/Ti1 : Gain  ParamDataTypeStr=double  OutDataTypeStr=double  SaturateOnIntegerOverflow=on
  Saturation2 : Saturate  UpperLimit=12  LowerLimit=0  OutDataTypeStr=double
  Sum1 : Sum  Inputs=+++  SaturateOnIntegerOverflow=on
  Sum4 : Sum  Inputs=-+  SaturateOnIntegerOverflow=on
  Unit Delay4 : UnitDelay  SampleTime=tsample
  kp2 : Gain  Gain=18*tsample  ParamDataTypeStr=double  OutDataTypeStr=double  SaturateOnIntegerOverflow=on
  ctrlv_out : Outport
  wires:
  ixi_tilde/1 -> 1/Ti1/1
  kp2/1 -> Sum1/2
  Sum4/1 -> Unit Delay4/1
  1/Ti/1 -> Sum1/1, Sum4/1
  Sum1/1 -> Saturation2/1
  Unit Delay4/1 -> Sum1/3
  Saturation2/1 -> ctrlv_out/1, Sum4/2
  1/Ti1/1 -> 1/Ti/1, kp2/1
